simulink model "zumo_control_distance_heading_mod"  (R2014b)
settings: Solver=ode3  SolverMode=SingleTasking  StartTime=0.0  StopTime=20  FixedStep=0.01  RelTol=1e-3
PreLoadFcn:
  | evalin('base','sim=1;');
  | evalin('base','control=0;');
  | evalin('base','bluetoothComm=0;');
  | prepareCurrentFolderForZumo;
  | load MagnetometerBus;
model workspace (MAT data in the model file):
  axleLength = Simulink.Parameter
  axleLength.Value = 9.8
  axleLength.Description = 'Distance between tire contact points
    | of the two wheels/treads
    | in units of centimeters.'
  axleLength.DataType = 'auto'
  commandPercmPerSecond = Simulink.Parameter
  commandPercmPerSecond.Value = 3.9547
  commandPercmPerSecond.Description = 'Convert units of ''command'' 
    | to units of ''cm/s''.
    | 
    | ''command'' is a value in the range [-256, 255].'
  commandPercmPerSecond.DataType = 'auto'
  symmetrizeMotors = Simulink.Parameter
  symmetrizeMotors.Value = 1
  symmetrizeMotors.Description = 'Scale one of the motor commands down 
    | (not up) to balance the motors. 
    | Once balanced, a value of x sent to either
    | motor will produce the same rate of rotation
    | in both motors.'
  symmetrizeMotors.DataType = 'auto'
  sampleTime = Simulink.Parameter
  sampleTime.Value = 0.01
  sampleTime.Description = 'Sample time (in seconds) of the trajectory simulator.'
  sampleTime.DataType = 'auto'
  commandThreshold = Simulink.Parameter
  commandThreshold.Value = 31.875
  commandThreshold.DataType = 'auto'
  lineThreshold = Simulink.Parameter
  lineThreshold.Value = 500
  lineThreshold.DataType = 'auto'
  velocity = Simulink.Parameter
  velocity.Value = 10
  velocity.Description = 'cm / s'
  velocity.DataType = 'auto'
  waveLength = Simulink.Parameter
  waveLength.Value = 8.6
  waveLength.Description = 'Units of cm.
    | 
    | The following condition must be satisfied: 
    | waveLength > 2*pi * velocity / sqrt(0.5 / sampleTime)
    | 
    | For reference,
    | robotLength = 8.6 cm
    | '
  waveLength.DataType = 'auto'
  compassBias = Simulink.Parameter
  compassBias.Value = 120
  compassBias.DataType = 'auto'
undefined symbols (not defined in the file or in its folder): magnitude
libraries: simulink x7, ZumoBotLib x2, arduinolib x2, etargetslib x2
settings Model: ExtModeTrigDuration=2  Creator=pkasseba  LastModifiedBy=sandip
settings DataIOCC: SignalLoggingSaveFormat=ModelDataLogs
settings OptimizationCC: OptimizeModelRefInitCode=on  LifeSpan=1
settings DebuggingCC: UnderspecifiedInitializationDetection=Classic  MergeDetectMultiDrivingBlocksExec=none  SolverPrmCheckMsg=none  MultiTaskDSMMsg=warning  MultiTaskCondExecSysMsg=none  StateNameClashWarn=warning
settings HardwareCC: ProdBitPerInt=16  ProdBitPerPointer=8  ProdIntDivRoundTo=Zero  ProdEndianess=LittleEndian  ProdWordSize=8  ProdHWDeviceType=Atmel->AVR
settings SFSimCC: SimParseCustomCode=off
settings RTWCC: SystemTargetFile=realtime.tlc  GenerateMakefile=off  TemplateMakefile=realtime.tmf  Description=Run on Target Hardware  RTWVerbose=off  ProcessScript=realtime_make_rtw_hook  IncludeERTFirstTime=on
settings STFCustomTargetCC: TargetLibSuffix=.a  GenerateSampleERTMain=on  ERTCustomFileBanners=on  SupportNonInlinedSFcns=off  SupportVariableSizeSignals=on  MATLABClassNameForMDSCustomization=Simulink.SoftwareTarget.ERTCustomization  GRTInterface=off  SystemTargetFile=realtime.tlc
settings ERTTargetCC: GenerateSampleERTMain=on  ParMdlRefBuildCompliant=off  CompOptLevelCompliant=off  ConcurrentExecutionCompliant=off  CombineOutputUpdateFcns=off  ERTFirstTimeCompliant=off  SupportContinuousTime=on  SupportVariableSizeSignals=on  ModelStepFunctionPrototypeControlCompliant=off  CPPClassGenCompliant=off  ExtModeTransport=3  ExtModeMexFile=ext_serial_win32_comm  ExtModeMexArgs=0 1 9600  InlinedParameterPlacement=NonHierarchical  ERTSrcFileBannerTemplate=realtime_code_template.cgt  ERTHdrFileBannerTemplate=realtime_code_template.cgt  ERTDataSrcFileTemplate=realtime_code_template.cgt  ERTDataHdrFileTemplate=realtime_code_template.cgt  ERTCustomFileTemplate=realtime_file_process.tlc

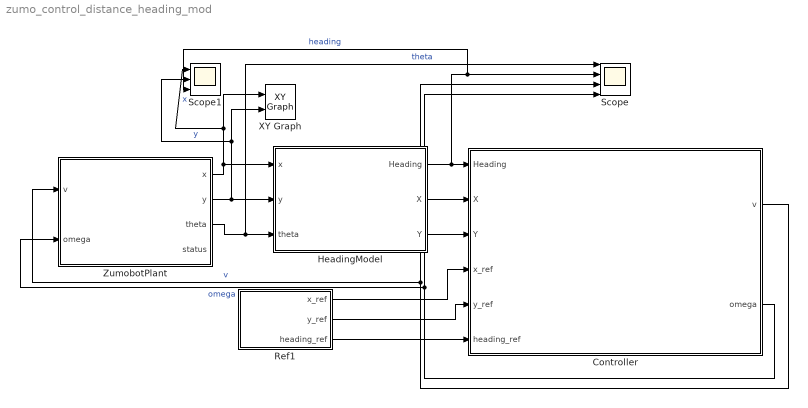
== system zumo_control_distance_heading_mod ==
  Controller : Subsystem
  HeadingModel : Subsystem  Variant=on
  Ref1 : Subsystem
  Scope : Scope  NumInputPorts=4
      settings: TimeRange=0.768348623853211  YMin=-2.5~184~14~-1  YMax=0~186.5~16~1  SaveName=ScopeData4
  Scope1 : Scope  NumInputPorts=3
      settings: YMin=180~100~0  YMax=340~240~350  SaveName=ScopeData2
  XY Graph : simulink/Sinks/XY Graph  xmin=-10  xmax=400  ymin=-10  ymax=400  st=-1
  ZumobotPlant : Subsystem  Variant=on
  wires:
  Controller/1(v) -> Scope/3, ZumobotPlant/1(v)  "v"
  Controller/2(omega) -> Scope/4, ZumobotPlant/2(omega)  "omega"
  ZumobotPlant/3(theta) -> Scope/1, HeadingModel/3(theta)  "theta"
  HeadingModel/2(X) -> Controller/2(X)
  HeadingModel/3(Y) -> Controller/3(Y)
  ZumobotPlant/1(x) -> Scope1/1, XY Graph/1, HeadingModel/1(x)  "x"
  ZumobotPlant/2(y) -> Scope1/2, XY Graph/2, HeadingModel/2(y)  "y"
  HeadingModel/1(Heading) -> Scope1/3, Scope/2, Controller/1(Heading)  "heading"
  Ref1/1(x_ref) -> Controller/4(x_ref)
  Ref1/2(y_ref) -> Controller/5(y_ref)
  Ref1/3(heading_ref) -> Controller/6(heading_ref)

== system zumo_control_distance_heading_mod/Controller ==
  Heading : Inport
  X : Inport  Port=2
  Y : Inport  Port=3
  x_ref : Inport  Port=4
  y_ref : Inport  Port=5
  heading_ref : Inport  Port=6
  Subsystem : Subsystem  Commented=on
  Subsystem1 : Subsystem  Commented=on
  Variant Subsystem : Subsystem  Variant=on
  v : Outport  InitialOutput=0
  omega : Outport  Port=2  InitialOutput=0
  wires:
  Y/1 -> Variant Subsystem/2(Y)
  Heading/1 -> Variant Subsystem/6(Heading)
  Variant Subsystem/1(v) -> v/1
  Variant Subsystem/2(omega) -> omega/1
  X/1 -> Variant Subsystem/1(X)
  x_ref/1 -> Variant Subsystem/3(DesiredX)
  y_ref/1 -> Variant Subsystem/4(DesiredY)
  heading_ref/1 -> Variant Subsystem/5(DesiredHeading)

== system zumo_control_distance_heading_mod/HeadingModel ==
  note: 1) Only subsystems can be added as variant choices at this level
      | 2) Blocks cannot be connected at this level as connectivity is
      | automatically determined at simulation, based on the active variant
  x : Inport
  y : Inport  Port=2
  theta : Inport  Port=3
  Simulation : Subsystem  VariantControl=sim==1
  Target : Subsystem  VariantControl=sim==0
  Heading : Outport
  X : Outport  Port=2
  Y : Outport  Port=3

== system zumo_control_distance_heading_mod/Ref1 ==
  DesiredHeading : Constant  Value=120
  DesiredX : Constant  Value=320
  DesiredY : Constant  Value=240
  x_ref : Outport
  y_ref : Outport  Port=2
  heading_ref : Outport  Port=3
  wires:
  DesiredX/1 -> x_ref/1
  DesiredY/1 -> y_ref/1
  DesiredHeading/1 -> heading_ref/1

== system zumo_control_distance_heading_mod/ZumobotPlant ==
  note: 1) Only subsystems can be added as variant choices at this level
      | 2) Blocks cannot be connected at this level as connectivity is
      | automatically determined at simulation, based on the active variant
  v : Inport
  omega : Inport  Port=2
  Simulation : Subsystem  VariantControl=sim==1
  Target : Subsystem  VariantControl=sim==0
  x : Outport
  y : Outport  Port=2
  theta : Outport  Port=3
  status : Outport  Port=4

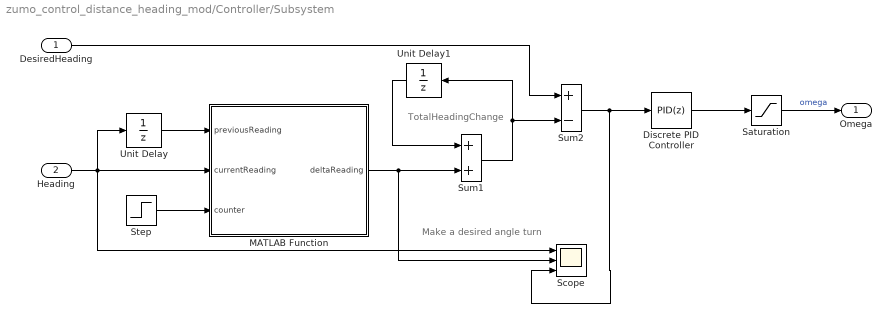
== system zumo_control_distance_heading_mod/Controller/Subsystem ==
  note: Make a desired angle turn
  note: TotalHeadingChange
  DesiredHeading : Inport
  Heading : Inport  Port=2
  Discrete PID Controller : simulink/Continuous/PID Controller  Controller=PID  TimeDomain=Discrete-time  SampleTime=0.01  IntegratorMethod=Forward Euler  FilterMethod=Forward Euler  Form=Parallel  P=20  I=0  D=0  N=100  InitialConditionSource=internal  InitialConditionForIntegrator=0  InitialConditionForFilter=0  ExternalReset=none  LimitOutput=off  UpperSaturationLimit=inf  LowerSaturationLimit=-inf  LinearizeAsGain=off  AntiWindupMode=none  Kb=1  TrackingMode=off  Kt=1  PParamMin=[]  PParamMax=[]  IParamMin=[]  IParamMax=[]  DParamMin=[]  DParamMax=[]  NParamMin=[]  NParamMax=[]  KbParamMin=[]  KbParamMax=[]  KtParamMin=[]  KtParamMax=[]  POutMin=[]  POutMax=[]  IOutMin=[]  IOutMax=[]  DOutMin=[]  DOutMax=[]  NOutMin=[]  NOutMax=[]  KbOutMin=[]  KbOutMax=[]  KtOutMin=[]  KtOutMax=[]  IntegratorOutMin=[]  IntegratorOutMax=[]  FilterOutMin=[]  FilterOutMax=[]  SumOutMin=[]  SumOutMax=[]  SumI1OutMin=[]  SumI1OutMax=[]  SumI2OutMin=[]  SumI2OutMax=[]  SumI3OutMin=[]  SumI3OutMax=[]  SumDOutMin=[]  SumDOutMax=[]  SaturationOutMin=[]  SaturationOutMax=[]  IntegratorContinuousStateAttributes=''  IntegratorStateMustResolveToSignalObject=off  IntegratorRTWStateStorageClass=Auto  FilterContinuousStateAttributes=''  FilterStateMustResolveToSignalObject=off  FilterRTWStateStorageClass=Auto
  MATLAB Function : MATLAB Function  TreatAsAtomicUnit=on
  Saturation : Saturate  UpperLimit=200  LowerLimit=0
  Scope : Scope  NumInputPorts=3
      settings: YMin=266~-1~-4  YMax=266~1~-4
  Step : Step  Time=2*sampleTime  SampleTime=sampleTime
  Sum1 : Sum
  Sum2 : Sum  Inputs=+-
  Unit Delay : UnitDelay  SampleTime=-1
  Unit Delay1 : UnitDelay  SampleTime=-1
  Omega : Outport
  wires:
  Sum1/1 -> Unit Delay1/1, Sum2/2
  Step/1 -> MATLAB Function/3(counter)
  MATLAB Function/1(deltaReading) -> Scope/2, Sum1/2
  Sum2/1 -> Discrete PID Controller/1, Scope/3
  Saturation/1 -> Omega/1  "omega"
  Unit Delay/1 -> MATLAB Function/1(previousReading)
  Unit Delay1/1 -> Sum1/1
  DesiredHeading/1 -> Sum2/1
  Heading/1 -> Unit Delay/1, MATLAB Function/2(currentReading), Scope/1
  Discrete PID Controller/1 -> Saturation/1

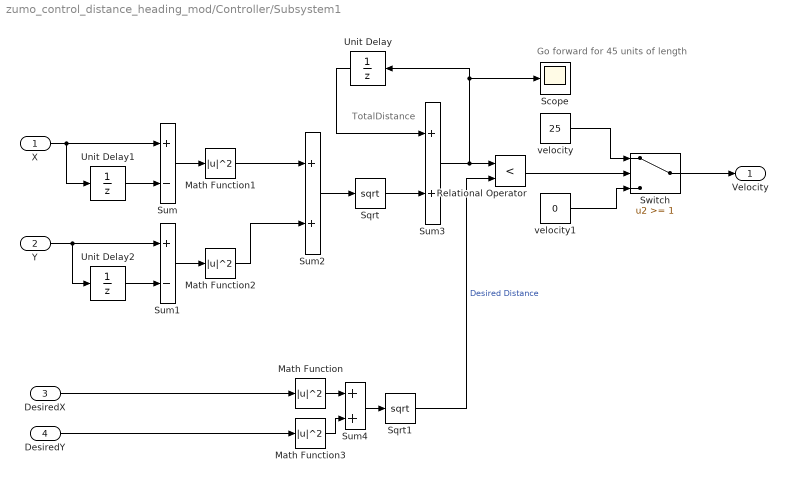
== system zumo_control_distance_heading_mod/Controller/Subsystem1 ==
  note: Go forward for 45 units of length
  note: TotalDistance
  X : Inport
  Y : Inport  Port=2
  DesiredX : Inport  Port=3
  DesiredY : Inport  Port=4
  Math Function{,1..3} (4 alike) : Math  Operator=magnitude^2  SaturateOnIntegerOverflow=on
  Relational Operator : RelationalOperator  Operator=<  OutDataTypeStr=boolean
  Scope : Scope
      settings: YMin=0  YMax=50
  Sqrt : Sqrt  SaturateOnIntegerOverflow=on
  Sqrt1 : Sqrt  SaturateOnIntegerOverflow=on
  Sum : Sum  Inputs=+-
  Sum1 : Sum  Inputs=+-
  Sum2 : Sum
  Sum3 : Sum
  Sum4 : Sum
  Switch : Switch  Threshold=1
  Unit Delay : UnitDelay  SampleTime=-1
  Unit Delay1 : UnitDelay  SampleTime=-1
  Unit Delay2 : UnitDelay  SampleTime=-1
  velocity : Constant  Value=25
  velocity1 : Constant  Value=0
  Velocity : Outport
  wires:
  X/1 -> Unit Delay1/1, Sum/1
  Sqrt/1 -> Sum3/2
  Sum/1 -> Math Function1/1
  Sum2/1 -> Sqrt/1
  Math Function1/1 -> Sum2/1
  velocity/1 -> Switch/1
  Unit Delay1/1 -> Sum/2
  Math Function2/1 -> Sum2/2
  Switch/1 -> Velocity/1
  Sum1/1 -> Math Function2/1
  Unit Delay2/1 -> Sum1/2
  Y/1 -> Unit Delay2/1, Sum1/1
  Unit Delay/1 -> Sum3/1
  Sum3/1 -> Relational Operator/1, Scope/1, Unit Delay/1
  velocity1/1 -> Switch/3
  Relational Operator/1 -> Switch/2
  Math Function3/1 -> Sum4/2
  Math Function/1 -> Sum4/1
  Sum4/1 -> Sqrt1/1
  Sqrt1/1 -> Relational Operator/2  "Desired Distance"
  DesiredX/1 -> Math Function/1
  DesiredY/1 -> Math Function3/1

== system zumo_control_distance_heading_mod/Controller/Variant Subsystem ==
  note: 1) Only subsystems can be added as variant choices at this level
      | 2) Blocks cannot be connected at this level as connectivity is
      | automatically determined at simulation, based on the active variant
  X : Inport
  Y : Inport  Port=2
  DesiredX : Inport  Port=3
  DesiredY : Inport  Port=4
  DesiredHeading : Inport  Port=5
  Heading : Inport  Port=6
  PrimitiveControl : Subsystem  VariantControl=control == 2
  controllyap : MATLAB Function  TreatAsAtomicUnit=on  VariantControl=control==0
  wmr : MATLAB Function  TreatAsAtomicUnit=on  VariantControl=control==1
  v : Outport
  omega : Outport  Port=2

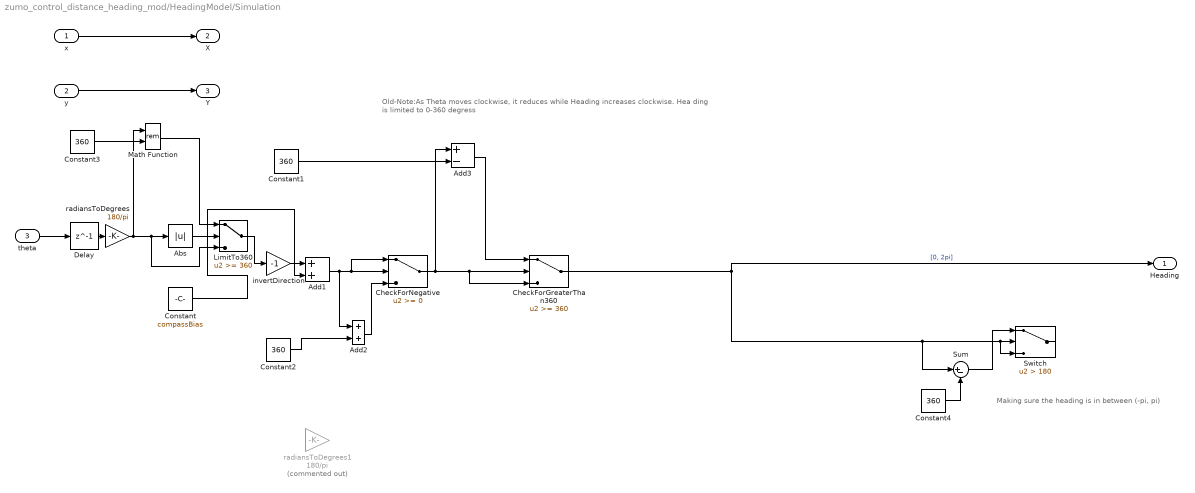
== system zumo_control_distance_heading_mod/HeadingModel/Simulation ==
  note: Old-Note:As Theta moves clockwise, it reduces while Heading increases clockwise.
      | Hea ding is limited to 0-360 degress
  note: Making sure the heading is in between (-pi, pi)
  x : Inport
  y : Inport  Port=2
  theta : Inport  Port=3
  Abs : Abs
  Add1 : Sum
  Add2 : Sum
  Add3 : Sum  Inputs=+-
  CheckForGreaterThan360 : Switch  Threshold=360
  CheckForNegative : Switch
  Constant : Constant  Value=compassBias
  Constant{1..4} (4 alike) : Constant  Value=360
  Delay : Delay  DelayLength=1  InitialCondition=0  SampleTime=sampleTime
  LimitTo360 : Switch  Threshold=360
  Math Function : Math  Operator=rem  SaturateOnIntegerOverflow=on
  Sum : Sum  Inputs=|+-
  Switch : Switch  Criteria=u2 > Threshold  Threshold=180
  invertDirection : Gain  Gain=-1
  radiansToDegrees : Gain  Gain=180/pi
  radiansToDegrees1 : Gain  Commented=on  Gain=180/pi
  Heading : Outport
  X : Outport  Port=2
  Y : Outport  Port=3
  wires:
  x/1 -> X/1
  y/1 -> Y/1
  Delay/1 -> radiansToDegrees/1
  Constant/1 -> Add1/2
  Constant1/1 -> Add3/2
  Add3/1 -> CheckForGreaterThan360/1
  invertDirection/1 -> Add1/1
  Add1/1 -> Add2/1, CheckForNegative/2, CheckForNegative/1
  CheckForNegative/1 -> CheckForGreaterThan360/3, CheckForGreaterThan360/2, Add3/1
  Constant2/1 -> Add2/2
  Add2/1 -> CheckForNegative/3
  radiansToDegrees/1 -> Math Function/1, LimitTo360/3, Abs/1
  LimitTo360/1 -> invertDirection/1
  Constant3/1 -> Math Function/2
  Math Function/1 -> LimitTo360/1
  Abs/1 -> LimitTo360/2
  CheckForGreaterThan360/1 -> Sum/1, Switch/3, Switch/2, Heading/1  "[0, 2pi]"
  Constant4/1 -> Sum/2
  theta/1 -> Delay/1
  Sum/1 -> Switch/1

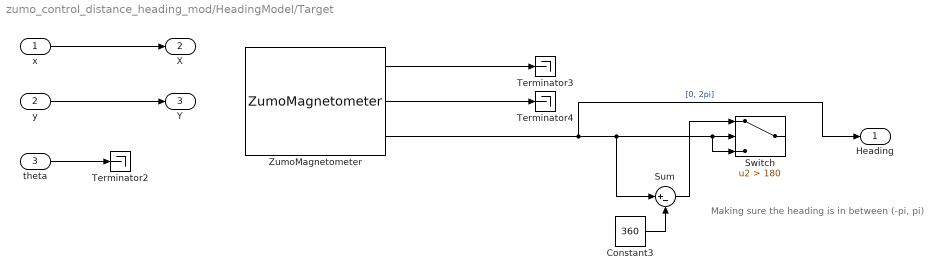
== system zumo_control_distance_heading_mod/HeadingModel/Target ==
  note: Making sure the heading is in between (-pi, pi)
  x : Inport
  y : Inport  Port=2
  theta : Inport  Port=3
  Constant3 : Constant  Value=360
  Sum : Sum  Inputs=|+-
  Switch : Switch  Criteria=u2 > Threshold  Threshold=180
  Terminator2 : Terminator
  Terminator3 : Terminator
  Terminator4 : Terminator
  ZumoMagnetometer : ZumoBotLib/ZumoMagnetometer  sampletime_lsm=0.01  debug_lsm=off  minX_lsm=-512  maxX_lsm=-279  minY_lsm=-163  maxY_lsm=99  minZ_lsm=1302  maxZ_lsm=1580
      link override S-Function Builder: Parameters=sampletime_lsm,boolean(debug_lsm),minX_lsm,maxX_lsm,minY_lsm,maxY_lsm,minZ_lsm,boolean(maxZ_lsm)
  Heading : Outport
  X : Outport  Port=2
  Y : Outport  Port=3
  wires:
  x/1 -> X/1
  y/1 -> Y/1
  theta/1 -> Terminator2/1
  ZumoMagnetometer/1 -> Terminator3/1
  ZumoMagnetometer/2 -> Terminator4/1
  ZumoMagnetometer/3 -> Heading/1, Sum/1, Switch/3, Switch/2  "[0, 2pi]"
  Constant3/1 -> Sum/2
  Sum/1 -> Switch/1

== system zumo_control_distance_heading_mod/ZumobotPlant/Simulation ==
  v : Inport
  omega : Inport  Port=2
  Computation of x,y,theta : Subsystem  Variant=on  OverrideUsingVariant=bluetoothComm==0
  Delay : Delay  DelayLength=1  InitialCondition=0
  degreesToRadians : Gain  Gain=pi/180
  motor command conversion : Subsystem
  x : Outport
  y : Outport  Port=2
  theta : Outport  Port=3
  status : Outport  Port=4
  wires:
  v/1 -> motor command conversion/1(v)
  Computation of x,y,theta/1(x) -> x/1
  Computation of x,y,theta/2(y) -> y/1
  omega/1 -> degreesToRadians/1
  Computation of x,y,theta/3(theta) -> theta/1
  degreesToRadians/1 -> motor command conversion/2(omega)
  motor command conversion/1(v_L v_R) -> Delay/1
  Delay/1 -> Computation of x,y,theta/1(v_L v_R)

== system zumo_control_distance_heading_mod/ZumobotPlant/Target ==
  v : Inport
  omega : Inport  Port=2
  Computation of x,y,theta : Subsystem  Variant=on  OverrideUsingVariant=bluetoothComm==1
  Demux : Demux  Outputs=2
  ZumoMotors : ZumoBotLib/ZumoMotors  flipLeft=off  flipRight=off
  degreesToRadians : Gain  Gain=pi/180
  motor command conversion : Subsystem
  x : Outport
  y : Outport  Port=2
  theta : Outport  Port=3
  status : Outport  Port=4
  wires:
  motor command conversion/1(v_L v_R) -> Computation of x,y,theta/1(v_L v_R), Demux/1
  Demux/1 -> ZumoMotors/1
  Demux/2 -> ZumoMotors/2
  v/1 -> motor command conversion/1(v)
  omega/1 -> degreesToRadians/1
  degreesToRadians/1 -> motor command conversion/2(omega)
  Computation of x,y,theta/1(x) -> x/1
  Computation of x,y,theta/2(y) -> y/1
  Computation of x,y,theta/3(theta) -> theta/1
  Computation of x,y,theta/4(status) -> status/1

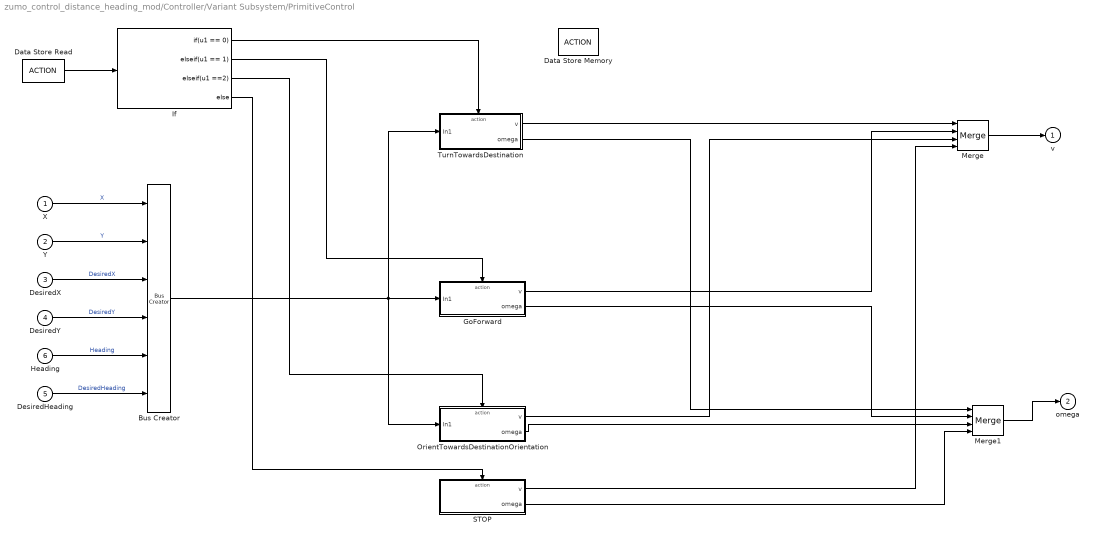
== system zumo_control_distance_heading_mod/Controller/Variant Subsystem/PrimitiveControl ==
  X : Inport
  Y : Inport  Port=2
  DesiredX : Inport  Port=3
  DesiredY : Inport  Port=4
  DesiredHeading : Inport  Port=5
  Heading : Inport  Port=6
  Bus Creator : BusCreator  Inputs=6
  Data Store Memory : DataStoreMemory  DataStoreName=ACTION  ReadBeforeWriteMsg=warning  WriteAfterWriteMsg=warning  WriteAfterReadMsg=warning
  Data Store Read : DataStoreRead  DialogController=Simulink.DDGSource  DataStoreName=ACTION  SampleTime=sampleTime  DataStoreElements=ACTION
  GoForward : Subsystem  TreatAsAtomicUnit=on
  If : If  IfExpression=u1 == 0  ElseIfExpressions=u1 == 1, u1 ==2
  Merge : Merge  Inputs=4
  Merge1 : Merge  Inputs=4
  OrientTowardsDestinationOrientation : Subsystem  TreatAsAtomicUnit=on
  STOP : Subsystem  TreatAsAtomicUnit=on
  TurnTowardsDestination : Subsystem  TreatAsAtomicUnit=on
  v : Outport
  omega : Outport  Port=2
  wires:
  X/1 -> Bus Creator/1  "X"
  Y/1 -> Bus Creator/2  "Y"
  DesiredX/1 -> Bus Creator/3  "DesiredX"
  DesiredY/1 -> Bus Creator/4  "DesiredY"
  DesiredHeading/1 -> Bus Creator/6  "DesiredHeading"
  Heading/1 -> Bus Creator/5  "Heading"
  Data Store Read/1 -> If/1
  If/1 -> TurnTowardsDestination/Action
  If/2 -> GoForward/Action
  If/3 -> OrientTowardsDestinationOrientation/Action
  Merge/1 -> v/1
  Merge1/1 -> omega/1
  TurnTowardsDestination/1(v) -> Merge/1
  GoForward/1(v) -> Merge/2
  OrientTowardsDestinationOrientation/1(v) -> Merge/3
  TurnTowardsDestination/2(omega) -> Merge1/1
  OrientTowardsDestinationOrientation/2(omega) -> Merge1/3
  GoForward/2(omega) -> Merge1/2
  Bus Creator/1 -> OrientTowardsDestinationOrientation/1(In1), TurnTowardsDestination/1(In1), GoForward/1(In1)
  STOP/1(v) -> Merge/4
  STOP/2(omega) -> Merge1/4
  If/4 -> STOP/Action

== system zumo_control_distance_heading_mod/ZumobotPlant/Simulation/Computation of x,y,theta ==
  note: 1) Only subsystems can be added as variant choices at this level
      | 2) Blocks cannot be connected at this level as connectivity is
      | automatically determined at simulation, based on the active variant
  v_L v_R : Inport
  simulated trajectory/ replacing encoders : Subsystem  VariantControl=bluetoothComm==0
  "values from bluetooth " : Subsystem  VariantControl=bluetoothComm==1
  x : Outport
  y : Outport  Port=2
  theta : Outport  Port=3

== system zumo_control_distance_heading_mod/ZumobotPlant/Simulation/motor command conversion ==
  note: or in matrix notation,
  note: v_L  = v - omega * axleLength/2
      | v_R = v + omega * axleLength/2
  note: [v_L; v_R] = [1 -axleLength/2; 1 axleLength/2] * [v; omega]
  v : Inport
  omega : Inport  Port=2
  Mux : Mux  Inputs=2
  Saturation [-256 255] : Saturate  UpperLimit=255  LowerLimit=-256
  change parameters : Gain  Gain=[1 -axleLength/2; 1 axleLength/2]  Multiplication=Matrix(K*u)
  change units : Gain  Gain=commandPercmPerSecond
  symmetrize motors : Gain  Gain=[1 symmetrizeMotors]
  v_L v_R : Outport
  wires:
  change parameters/1 -> symmetrize motors/1  "v_L v_R"
  change units/1 -> Saturation [-256 255]/1  "v_L v_R (command)"
  symmetrize motors/1 -> change units/1  "v_L v_R (cm/s)"
  Saturation [-256 255]/1 -> v_L v_R/1
  Mux/1 -> change parameters/1
  omega/1 -> Mux/2
  v/1 -> Mux/1

== system zumo_control_distance_heading_mod/ZumobotPlant/Target/Computation of x,y,theta ==
  note: 1) Only subsystems can be added as variant choices at this level
      | 2) Blocks cannot be connected at this level as connectivity is
      | automatically determined at simulation, based on the active variant
  v_L v_R : Inport
  simulated trajectory/ replacing encoders : Subsystem  VariantControl=bluetoothComm==0
  "values from bluetooth " : Subsystem  VariantControl=bluetoothComm==1
  x : Outport
  y : Outport  Port=2
  theta : Outport  Port=3
  status : Outport  Port=4

== system zumo_control_distance_heading_mod/ZumobotPlant/Target/motor command conversion ==
  note: or in matrix notation,
  note: v_L  = v - omega * axleLength/2
      | v_R = v + omega * axleLength/2
  note: [v_L; v_R] = [1 -axleLength/2; 1 axleLength/2] * [v; omega]
  v : Inport
  omega : Inport  Port=2
  Mux : Mux  Inputs=2
  Saturation [-256 255] : Saturate  UpperLimit=255  LowerLimit=-256
  change parameters : Gain  Gain=[1 -axleLength/2; 1 axleLength/2]  Multiplication=Matrix(K*u)
  change units : Gain  Gain=commandPercmPerSecond
  scaling to +/-50 : Lookup_n-D  Commented=through  NumberOfTableDimensions=1  BreakpointsForDimension1=[-500 -256 255 500]  Table=[-70 -70 70 70]  ExtrapMethod=Clip  InternalRulePriority=Speed  RndMeth=Simplest  InputSameDT=on
  symmetrize motors : Gain  Gain=[1 symmetrizeMotors]
  v_L v_R : Outport
  wires:
  change parameters/1 -> symmetrize motors/1  "v_L v_R"
  change units/1 -> Saturation [-256 255]/1  "v_L v_R (command)"
  symmetrize motors/1 -> change units/1  "v_L v_R (cm/s)"
  Saturation [-256 255]/1 -> scaling to +/-50/1
  Mux/1 -> change parameters/1
  omega/1 -> Mux/2
  v/1 -> Mux/1
  scaling to +/-50/1 -> v_L v_R/1

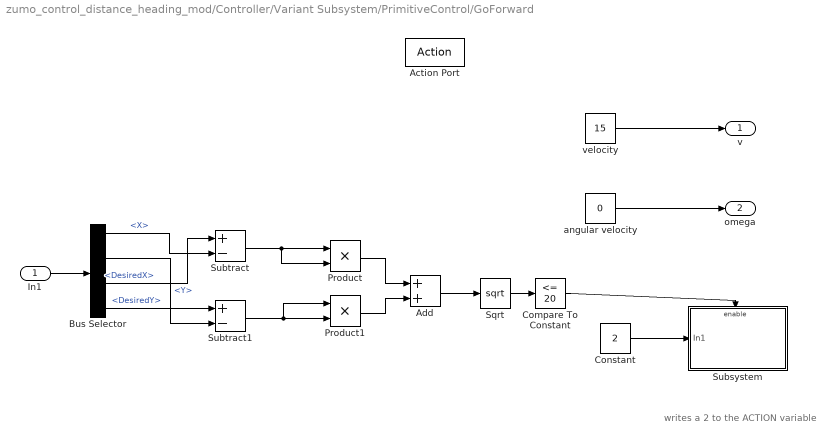
== system zumo_control_distance_heading_mod/Controller/Variant Subsystem/PrimitiveControl/GoForward ==
  note: writes a 2 to the ACTION variable
  In1 : Inport
  Action Port : ActionPort  ActionType=elseif
  Add : Sum
  Bus Selector : BusSelector  OutputSignals=X,Y,DesiredX,DesiredY
  Compare To Constant : simulink/Logic and Bit Operations/Compare To Constant  relop=<=  const=20  OutDataTypeStr=boolean
  Constant : Constant  Value=2
  Product : Product
  Product1 : Product
  Sqrt : Sqrt  SaturateOnIntegerOverflow=on
  Subsystem : Subsystem
  Subtract : Sum  Inputs=+-
  Subtract1 : Sum  Inputs=+-
  angular velocity : Constant  Value=0
  velocity : Constant  Value=15
  v : Outport  InitialOutput=0
  omega : Outport  Port=2  InitialOutput=0
  wires:
  angular velocity/1 -> omega/1
  velocity/1 -> v/1
  In1/1 -> Bus Selector/1
  Add/1 -> Sqrt/1
  Product/1 -> Add/1
  Product1/1 -> Add/2
  Subtract/1 -> Product/2, Product/1
  Subtract1/1 -> Product1/2, Product1/1
  Bus Selector/1 -> Subtract/2  "<X>"
  Bus Selector/3 -> Subtract/1  "<DesiredX>"
  Bus Selector/2 -> Subtract1/2  "<Y>"
  Bus Selector/4 -> Subtract1/1  "<DesiredY>"
  Sqrt/1 -> Compare To Constant/1
  Compare To Constant/1 -> Subsystem/Enable
  Constant/1 -> Subsystem/1(In1)

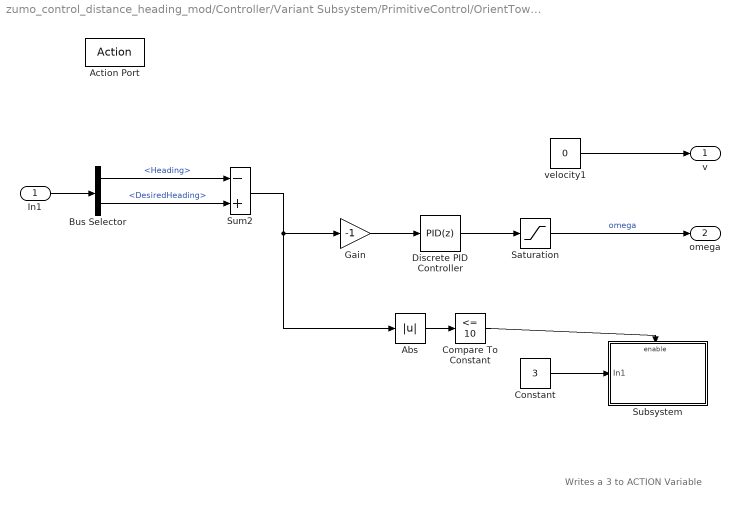
== system zumo_control_distance_heading_mod/Controller/Variant Subsystem/PrimitiveControl/OrientTowardsDestinationOrientation ==
  note: Writes a 3 to ACTION Variable
  In1 : Inport
  Action Port : ActionPort  ActionType=elseif
  Abs : Abs
  Bus Selector : BusSelector  OutputSignals=Heading,DesiredHeading
  Compare To Constant : simulink/Logic and Bit Operations/Compare To Constant  relop=<=  const=10  OutDataTypeStr=boolean
  Constant : Constant  Value=3
  Discrete PID Controller : simulink/Continuous/PID Controller  Controller=PID  TimeDomain=Discrete-time  SampleTime=0.01  IntegratorMethod=Forward Euler  FilterMethod=Forward Euler  Form=Parallel  P=100  I=0  D=0  N=100  InitialConditionSource=internal  InitialConditionForIntegrator=0  InitialConditionForFilter=0  ExternalReset=none  LimitOutput=off  UpperSaturationLimit=inf  LowerSaturationLimit=-inf  LinearizeAsGain=off  AntiWindupMode=none  Kb=1  TrackingMode=off  Kt=1  PParamMin=[]  PParamMax=[]  IParamMin=[]  IParamMax=[]  DParamMin=[]  DParamMax=[]  NParamMin=[]  NParamMax=[]  KbParamMin=[]  KbParamMax=[]  KtParamMin=[]  KtParamMax=[]  POutMin=[]  POutMax=[]  IOutMin=[]  IOutMax=[]  DOutMin=[]  DOutMax=[]  NOutMin=[]  NOutMax=[]  KbOutMin=[]  KbOutMax=[]  KtOutMin=[]  KtOutMax=[]  IntegratorOutMin=[]  IntegratorOutMax=[]  FilterOutMin=[]  FilterOutMax=[]  SumOutMin=[]  SumOutMax=[]  SumI1OutMin=[]  SumI1OutMax=[]  SumI2OutMin=[]  SumI2OutMax=[]  SumI3OutMin=[]  SumI3OutMax=[]  SumDOutMin=[]  SumDOutMax=[]  SaturationOutMin=[]  SaturationOutMax=[]  IntegratorContinuousStateAttributes=''  IntegratorStateMustResolveToSignalObject=off  IntegratorRTWStateStorageClass=Auto  FilterContinuousStateAttributes=''  FilterStateMustResolveToSignalObject=off  FilterRTWStateStorageClass=Auto  DifferentiatorICPrevScaledInput=0  DifferentiatorOutMin=[]  DifferentiatorOutMax=[]  UseFilter=on
  Gain : Gain  Gain=-1
  Saturation : Saturate  UpperLimit=100  LowerLimit=-100
  Subsystem : Subsystem
  Sum2 : Sum  Inputs=-+
  velocity1 : Constant  Value=0
  v : Outport
  omega : Outport  Port=2
  wires:
  In1/1 -> Bus Selector/1
  velocity1/1 -> v/1
  Bus Selector/2 -> Sum2/2  "<DesiredHeading>"
  Sum2/1 -> Abs/1, Gain/1
  Saturation/1 -> omega/1  "omega"
  Bus Selector/1 -> Sum2/1  "<Heading>"
  Discrete PID Controller/1 -> Saturation/1
  Abs/1 -> Compare To Constant/1
  Compare To Constant/1 -> Subsystem/Enable
  Constant/1 -> Subsystem/1(In1)
  Gain/1 -> Discrete PID Controller/1

== system zumo_control_distance_heading_mod/Controller/Variant Subsystem/PrimitiveControl/STOP ==
  Action Port : ActionPort  ActionType=else
  velocity1 : Constant  Value=0
  velocity2 : Constant  Value=0
  v : Outport
  omega : Outport  Port=2
  wires:
  velocity1/1 -> v/1
  velocity2/1 -> omega/1

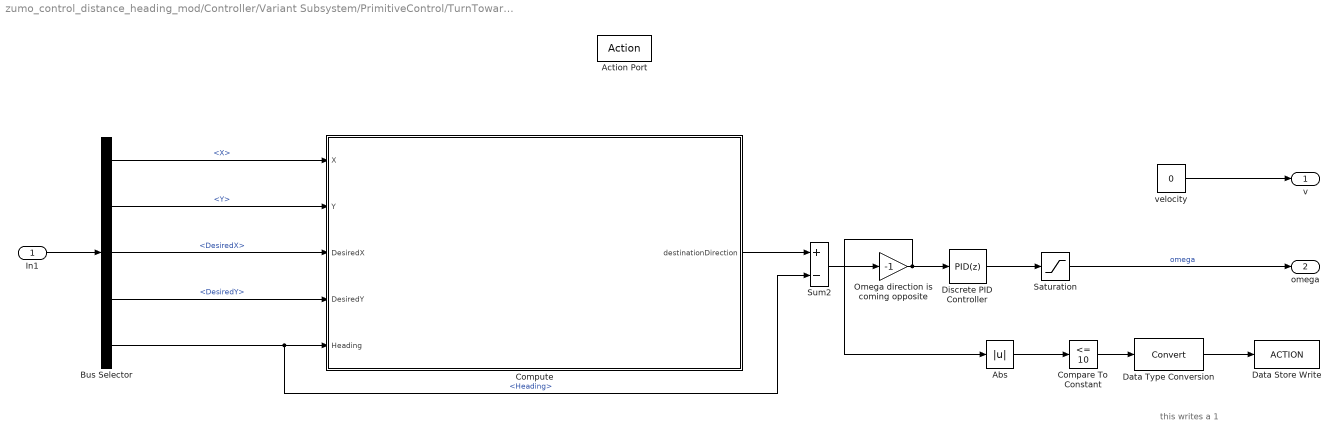
== system zumo_control_distance_heading_mod/Controller/Variant Subsystem/PrimitiveControl/TurnTowardsDestination ==
  note: this writes a 1
  In1 : Inport
  Action Port : ActionPort  ActionType=then
  Abs : Abs
  Bus Selector : BusSelector  OutputSignals=X,Y,DesiredX,DesiredY,Heading
  Compare To Constant : simulink/Logic and Bit Operations/Compare To Constant  relop=<=  const=10  OutDataTypeStr=boolean
  Compute : MATLAB Function  TreatAsAtomicUnit=on
  Data Store Write : DataStoreWrite  DialogController=Simulink.DDGSource  DataStoreName=ACTION  DataStoreElements=ACTION
  Data Type Conversion : DataTypeConversion
  Discrete PID Controller : simulink/Continuous/PID Controller  Controller=PID  TimeDomain=Discrete-time  SampleTime=0.01  IntegratorMethod=Forward Euler  FilterMethod=Forward Euler  Form=Parallel  P=100  I=0  D=0  N=100  InitialConditionSource=internal  InitialConditionForIntegrator=0  InitialConditionForFilter=0  ExternalReset=none  LimitOutput=off  UpperSaturationLimit=inf  LowerSaturationLimit=-inf  LinearizeAsGain=off  AntiWindupMode=none  Kb=1  TrackingMode=off  Kt=1  PParamMin=[]  PParamMax=[]  IParamMin=[]  IParamMax=[]  DParamMin=[]  DParamMax=[]  NParamMin=[]  NParamMax=[]  KbParamMin=[]  KbParamMax=[]  KtParamMin=[]  KtParamMax=[]  POutMin=[]  POutMax=[]  IOutMin=[]  IOutMax=[]  DOutMin=[]  DOutMax=[]  NOutMin=[]  NOutMax=[]  KbOutMin=[]  KbOutMax=[]  KtOutMin=[]  KtOutMax=[]  IntegratorOutMin=[]  IntegratorOutMax=[]  FilterOutMin=[]  FilterOutMax=[]  SumOutMin=[]  SumOutMax=[]  SumI1OutMin=[]  SumI1OutMax=[]  SumI2OutMin=[]  SumI2OutMax=[]  SumI3OutMin=[]  SumI3OutMax=[]  SumDOutMin=[]  SumDOutMax=[]  SaturationOutMin=[]  SaturationOutMax=[]  IntegratorContinuousStateAttributes=''  IntegratorStateMustResolveToSignalObject=off  IntegratorRTWStateStorageClass=Auto  FilterContinuousStateAttributes=''  FilterStateMustResolveToSignalObject=off  FilterRTWStateStorageClass=Auto  DifferentiatorICPrevScaledInput=0  DifferentiatorOutMin=[]  DifferentiatorOutMax=[]  UseFilter=on
  Omega direction is coming opposite : Gain  Gain=-1
  Saturation : Saturate  UpperLimit=100  LowerLimit=-100
  Sum2 : Sum  Inputs=+-
  velocity : Constant  Value=0
  v : Outport  InitialOutput=0
  omega : Outport  Port=2
  wires:
  velocity/1 -> v/1
  In1/1 -> Bus Selector/1
  Bus Selector/1 -> Compute/1(X)  "<X>"
  Bus Selector/2 -> Compute/2(Y)  "<Y>"
  Bus Selector/3 -> Compute/3(DesiredX)  "<DesiredX>"
  Bus Selector/4 -> Compute/4(DesiredY)  "<DesiredY>"
  Bus Selector/5 -> Sum2/2, Compute/5(Heading)  "<Heading>"
  Sum2/1 -> Omega direction is coming opposite/1
  Saturation/1 -> omega/1  "omega"
  Compute/1(destinationDirection) -> Sum2/1
  Discrete PID Controller/1 -> Saturation/1
  Abs/1 -> Compare To Constant/1
  Compare To Constant/1 -> Data Type Conversion/1
  Data Type Conversion/1 -> Data Store Write/1
  Omega direction is coming opposite/1 -> Abs/1, Discrete PID Controller/1

== system zumo_control_distance_heading_mod/ZumobotPlant/Simulation/Computation of x,y,theta/simulated trajectory// replacing encoders ==
  v_L v_R : Inport
  Delay : Delay  DelayLength=1  InitialCondition=0
  Demux : Demux  Outputs=2
  Effective Motor Command : Subsystem
  Scope : Scope  NumInputPorts=2
      settings: YMin=-1~0.188496  YMax=1~0.188496  SaveName=ScopeData3
  calculate simulated trajectory1 : Subsystem
  change parameters : Gain  Gain=[0.5 0.5; -1/axleLength 1/axleLength]  Multiplication=Matrix(K*u)
  change units : Gain  Gain=1/commandPercmPerSecond
  x : Outport
  y : Outport  Port=2
  theta : Outport  Port=3
  wires:
  Demux/2 -> Scope/1, calculate simulated trajectory1/2(omega)
  Demux/1 -> calculate simulated trajectory1/1(v)
  v_L v_R/1 -> Delay/1
  Effective Motor Command/1(c_eff) -> change units/1  "v_L v_R (command)"
  change units/1 -> change parameters/1  "v_L v_R (cm/s)"
  change parameters/1 -> Demux/1  "v omega"
  calculate simulated trajectory1/2(y) -> y/1
  calculate simulated trajectory1/1(x) -> x/1
  calculate simulated trajectory1/3(theta) -> Scope/2, theta/1
  Delay/1 -> Effective Motor Command/1(c)

== system zumo_control_distance_heading_mod/ZumobotPlant/Simulation/Computation of x,y,theta/values from bluetooth  ==
  v_L v_R : Inport
  Serial Receive : arduinolib/Serial Receive  portNumber=0  showOutStatus=on  sampleTime=1  blockPlatform=arduino
  Subsystem : Subsystem
  Subsystem1 : Subsystem
  Terminator : Terminator
  x : Outport
  y : Outport  Port=2
  theta : Outport  Port=3
  wires:
  v_L v_R/1 -> Terminator/1
  Subsystem/1(Out1) -> x/1
  Subsystem/2(Out2) -> y/1
  Subsystem/3(Out3) -> theta/1
  Serial Receive/1 -> Subsystem1/1(In1)  "[x,y]"
  Subsystem1/1(Out1) -> Subsystem/1(In1)
  Subsystem1/2(status) -> Subsystem/Trigger
  Serial Receive/2 -> Subsystem1/Trigger

== system zumo_control_distance_heading_mod/ZumobotPlant/Target/Computation of x,y,theta/simulated trajectory// replacing encoders ==
  v_L v_R : Inport
  Delay : Delay  DelayLength=1  InitialCondition=0
  Demux : Demux  Outputs=2
  Effective Motor Command : Subsystem
  Scope : Scope  NumInputPorts=2
      settings: YMin=-1~0.188496  YMax=1~0.188496  SaveName=ScopeData3
  calculate simulated trajectory1 : Subsystem
  change parameters : Gain  Gain=[0.5 0.5; -1/axleLength 1/axleLength]  Multiplication=Matrix(K*u)
  change units : Gain  Gain=1/commandPercmPerSecond
  x : Outport
  y : Outport  Port=2
  theta : Outport  Port=3
  status : Outport  Port=4
  wires:
  Demux/2 -> Scope/1, calculate simulated trajectory1/2(omega)
  Demux/1 -> calculate simulated trajectory1/1(v)
  v_L v_R/1 -> Delay/1
  Effective Motor Command/1(c_eff) -> change units/1  "v_L v_R (command)"
  change units/1 -> change parameters/1  "v_L v_R (cm/s)"
  change parameters/1 -> Demux/1  "v omega"
  calculate simulated trajectory1/2(y) -> y/1
  calculate simulated trajectory1/1(x) -> x/1
  calculate simulated trajectory1/3(theta) -> Scope/2, theta/1
  Delay/1 -> Effective Motor Command/1(c)

== system zumo_control_distance_heading_mod/ZumobotPlant/Target/Computation of x,y,theta/values from bluetooth  ==
  v_L v_R : Inport
  Serial Receive : arduinolib/Serial Receive  portNumber=0  showOutStatus=on  sampleTime=0.01  blockPlatform=arduino
  Subsystem : Subsystem
  Subsystem1 : Subsystem
  Terminator : Terminator
  x : Outport
  y : Outport  Port=2
  theta : Outport  Port=3
  status : Outport  Port=4
  wires:
  v_L v_R/1 -> Terminator/1
  Subsystem/3(theta) -> theta/1
  Serial Receive/1 -> Subsystem1/1(In1)  "[x,y]"
  Subsystem1/1(Out1) -> Subsystem/1(In1)
  Subsystem/1(x) -> x/1
  Subsystem/2(y) -> y/1
  Subsystem1/2(status) -> Subsystem/Enable, status/1
  Serial Receive/2 -> Subsystem1/Enable

== system zumo_control_distance_heading_mod/Controller/Variant Subsystem/PrimitiveControl/GoForward/Subsystem ==
  In1 : Inport
  Enable : EnablePort
  Data Store Write : DataStoreWrite  DialogController=Simulink.DDGSource  DataStoreName=ACTION  DataStoreElements=ACTION
  wires:
  In1/1 -> Data Store Write/1

== system zumo_control_distance_heading_mod/Controller/Variant Subsystem/PrimitiveControl/OrientTowardsDestinationOrientation/Subsystem ==
  In1 : Inport
  Enable : EnablePort
  Data Store Write : DataStoreWrite  DialogController=Simulink.DDGSource  DataStoreName=ACTION  DataStoreElements=ACTION
  wires:
  In1/1 -> Data Store Write/1

== system zumo_control_distance_heading_mod/ZumobotPlant/Simulation/Computation of x,y,theta/simulated trajectory// replacing encoders/Effective Motor Command ==
  note: Zumobot does not move when given a command
      | with an abs less than 50 on a smooth surface,
      | so such commands are effectively 0.
  note: Do not saturate this signal.The process of symmetrizing
      | the motor commands gives rise to this artificial signal,
      | which can exceed the value of 255.
  c : Inport
  Abs : Abs
  Constant1 : Constant  Value=0
  Sum : Sum  Inputs=|+-
  Switch : Switch
  command threshold : Constant  Value=commandThreshold
  symmetrize motors : Gain  Gain=[1 1/symmetrizeMotors]
  c_eff : Outport
  wires:
  Switch/1 -> c_eff/1
  symmetrize motors/1 -> Abs/1, Switch/1
  Sum/1 -> Switch/2
  Abs/1 -> Sum/1
  command threshold/1 -> Sum/2
  c/1 -> symmetrize motors/1  "v_L v_R"
  Constant1/1 -> Switch/3

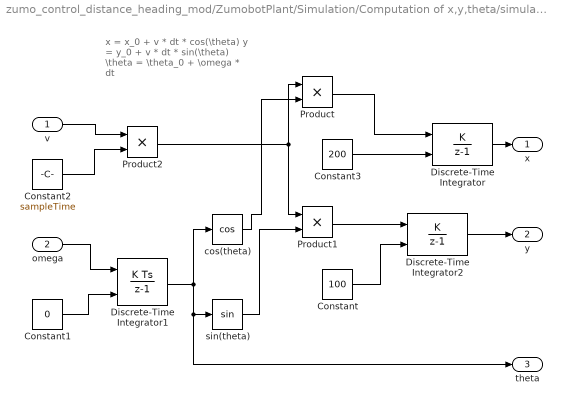
== system zumo_control_distance_heading_mod/ZumobotPlant/Simulation/Computation of x,y,theta/simulated trajectory// replacing encoders/calculate simulated trajectory1 ==
  note: x = x_0 + v * dt * cos(\theta)
      | y = y_0 + v * dt * sin(\theta)
      | \theta = \theta_0 + \omega * dt
  v : Inport
  omega : Inport  Port=2
  Constant : Constant  Value=100
  Constant1 : Constant  Value=0
  Constant2 : Constant  Value=sampleTime
  Constant3 : Constant  Value=200
  Discrete-Time Integrator : DiscreteIntegrator  IntegratorMethod=Accumulation: Forward Euler  InitialConditionSource=external  SampleTime=-1
  Discrete-Time Integrator1 : DiscreteIntegrator  InitialConditionSource=external  SampleTime=-1
  Discrete-Time Integrator2 : DiscreteIntegrator  IntegratorMethod=Accumulation: Forward Euler  InitialConditionSource=external  SampleTime=-1
  Product : Product
  Product1 : Product
  Product2 : Product
  cos(theta) : Trigonometry  Operator=cos
  sin(theta) : Trigonometry
  x : Outport
  y : Outport  Port=2
  theta : Outport  Port=3
  wires:
  omega/1 -> Discrete-Time Integrator1/1
  v/1 -> Product2/1
  Discrete-Time Integrator1/1 -> theta/1, sin(theta)/1, cos(theta)/1
  Product/1 -> Discrete-Time Integrator/1
  cos(theta)/1 -> Product/2
  Product2/1 -> Product/1, Product1/1
  sin(theta)/1 -> Product1/2
  Constant3/1 -> Discrete-Time Integrator/2
  Constant1/1 -> Discrete-Time Integrator1/2
  Constant2/1 -> Product2/2
  Discrete-Time Integrator/1 -> x/1
  Product1/1 -> Discrete-Time Integrator2/1
  Discrete-Time Integrator2/1 -> y/1
  Constant/1 -> Discrete-Time Integrator2/2

== system zumo_control_distance_heading_mod/ZumobotPlant/Simulation/Computation of x,y,theta/values from bluetooth /Subsystem ==
  In1 : Inport
  Trigger : TriggerPort  PortDimensions=1
  Byte Unpack : etargetslib/Byte Unpack  dimensions={1,1}  datatypes={'uint16', 'uint16'}  byteAlign=1
  Fcn : Fcn  Expr=atan2(u(1), u(2))
  Mux : Mux  Inputs=2
  Subtract : Sum  Inputs=+-
  Subtract1 : Sum  Inputs=+-
  Unit Delay : UnitDelay  SampleTime=-1
  Unit Delay1 : UnitDelay  SampleTime=-1
  Out1 : Outport
  Out2 : Outport  Port=2
  Out3 : Outport  Port=3
  wires:
  Byte Unpack/1 -> Unit Delay/1, Out1/1, Subtract/1
  Byte Unpack/2 -> Unit Delay1/1, Out2/1, Subtract1/1
  Subtract1/1 -> Mux/2  "dy"
  Mux/1 -> Fcn/1
  Subtract/1 -> Mux/1  "dx"
  Fcn/1 -> Out3/1
  Unit Delay/1 -> Subtract/2
  Unit Delay1/1 -> Subtract1/2
  In1/1 -> Byte Unpack/1

== system zumo_control_distance_heading_mod/ZumobotPlant/Simulation/Computation of x,y,theta/values from bluetooth /Subsystem1 ==
  In1 : Inport
  Trigger : TriggerPort  PortDimensions=1
  MATLAB Function : MATLAB Function  TreatAsAtomicUnit=on
  Out1 : Outport
  status : Outport  Port=2
  wires:
  In1/1 -> MATLAB Function/1(u)
  MATLAB Function/1(y) -> Out1/1
  MATLAB Function/2(trigger) -> status/1

== system zumo_control_distance_heading_mod/ZumobotPlant/Target/Computation of x,y,theta/simulated trajectory// replacing encoders/Effective Motor Command ==
  note: Zumobot does not move when given a command
      | with an abs less than 50 on a smooth surface,
      | so such commands are effectively 0.
  note: Do not saturate this signal.The process of symmetrizing
      | the motor commands gives rise to this artificial signal,
      | which can exceed the value of 255.
  c : Inport
  Abs : Abs
  Constant1 : Constant  Value=0
  Sum : Sum  Inputs=|+-
  Switch : Switch
  command threshold : Constant  Value=commandThreshold
  symmetrize motors : Gain  Gain=[1 1/symmetrizeMotors]
  c_eff : Outport
  wires:
  Switch/1 -> c_eff/1
  symmetrize motors/1 -> Abs/1, Switch/1
  Sum/1 -> Switch/2
  Abs/1 -> Sum/1
  command threshold/1 -> Sum/2
  c/1 -> symmetrize motors/1  "v_L v_R"
  Constant1/1 -> Switch/3

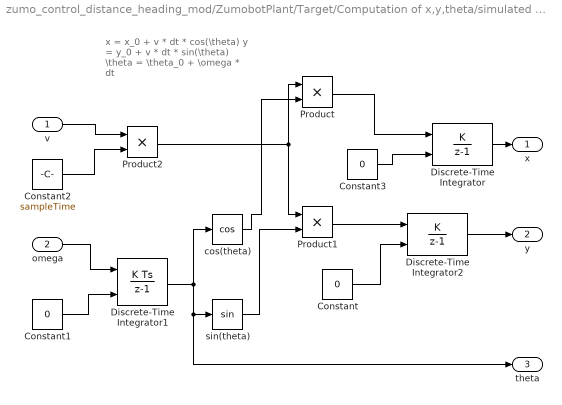
== system zumo_control_distance_heading_mod/ZumobotPlant/Target/Computation of x,y,theta/simulated trajectory// replacing encoders/calculate simulated trajectory1 ==
  note: x = x_0 + v * dt * cos(\theta)
      | y = y_0 + v * dt * sin(\theta)
      | \theta = \theta_0 + \omega * dt
  v : Inport
  omega : Inport  Port=2
  Constant : Constant  Value=0
  Constant1 : Constant  Value=0
  Constant2 : Constant  Value=sampleTime
  Constant3 : Constant  Value=0
  Discrete-Time Integrator : DiscreteIntegrator  IntegratorMethod=Accumulation: Forward Euler  InitialConditionSource=external  SampleTime=-1
  Discrete-Time Integrator1 : DiscreteIntegrator  InitialConditionSource=external  SampleTime=-1
  Discrete-Time Integrator2 : DiscreteIntegrator  IntegratorMethod=Accumulation: Forward Euler  InitialConditionSource=external  SampleTime=-1
  Product : Product
  Product1 : Product
  Product2 : Product
  cos(theta) : Trigonometry  Operator=cos
  sin(theta) : Trigonometry
  x : Outport
  y : Outport  Port=2
  theta : Outport  Port=3
  wires:
  omega/1 -> Discrete-Time Integrator1/1
  v/1 -> Product2/1
  Discrete-Time Integrator1/1 -> theta/1, sin(theta)/1, cos(theta)/1
  Product/1 -> Discrete-Time Integrator/1
  cos(theta)/1 -> Product/2
  Product2/1 -> Product/1, Product1/1
  sin(theta)/1 -> Product1/2
  Constant3/1 -> Discrete-Time Integrator/2
  Constant1/1 -> Discrete-Time Integrator1/2
  Constant2/1 -> Product2/2
  Discrete-Time Integrator/1 -> x/1
  Product1/1 -> Discrete-Time Integrator2/1
  Discrete-Time Integrator2/1 -> y/1
  Constant/1 -> Discrete-Time Integrator2/2

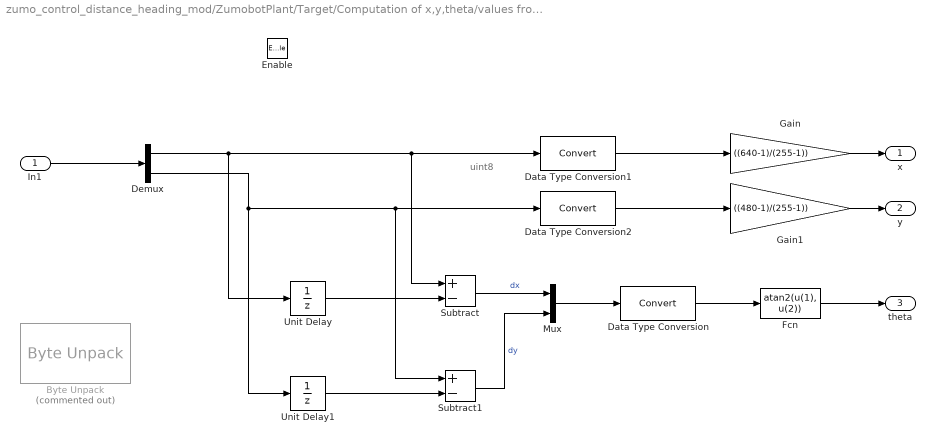
== system zumo_control_distance_heading_mod/ZumobotPlant/Target/Computation of x,y,theta/values from bluetooth /Subsystem ==
  note: uint8
  In1 : Inport
  Enable : EnablePort
  Byte Unpack : etargetslib/Byte Unpack  Commented=on  dimensions={1,1}  datatypes={'uint16', 'uint16'}  byteAlign=1
  Data Type Conversion : DataTypeConversion
  Data Type Conversion1 : DataTypeConversion
  Data Type Conversion2 : DataTypeConversion
  Demux : Demux  Outputs=2
  Fcn : Fcn  Expr=atan2(u(1), u(2))
  Gain : Gain  Gain=((640-1)/(255-1))
  Gain1 : Gain  Gain=((480-1)/(255-1))
  Mux : Mux  Inputs=2
  Subtract : Sum  Inputs=+-
  Subtract1 : Sum  Inputs=+-
  Unit Delay : UnitDelay  SampleTime=-1
  Unit Delay1 : UnitDelay  SampleTime=-1
  x : Outport  InitialOutput=150
  y : Outport  Port=2  InitialOutput=150
  theta : Outport  Port=3
  wires:
  Demux/1 -> Unit Delay/1, Data Type Conversion1/1, Subtract/1
  Demux/2 -> Unit Delay1/1, Data Type Conversion2/1, Subtract1/1
  Subtract1/1 -> Mux/2  "dy"
  Mux/1 -> Data Type Conversion/1
  Subtract/1 -> Mux/1  "dx"
  Fcn/1 -> theta/1
  Unit Delay/1 -> Subtract/2
  Unit Delay1/1 -> Subtract1/2
  In1/1 -> Demux/1
  Data Type Conversion/1 -> Fcn/1
  Data Type Conversion1/1 -> Gain/1
  Data Type Conversion2/1 -> Gain1/1
  Gain/1 -> x/1
  Gain1/1 -> y/1

== system zumo_control_distance_heading_mod/ZumobotPlant/Target/Computation of x,y,theta/values from bluetooth /Subsystem1 ==
  In1 : Inport
  Enable : EnablePort
  MATLAB Function : MATLAB Function  TreatAsAtomicUnit=on
  Out1 : Outport
  status : Outport  Port=2
  wires:
  In1/1 -> MATLAB Function/1(u)
  MATLAB Function/1(y) -> Out1/1
  MATLAB Function/2(trigger) -> status/1

== matlab function zumo_control_distance_heading_mod/ZumobotPlant/Target/Computation of x,y,theta/values from bluetooth /Subsystem1/MATLAB Function ==
  data: u input; y output; trigger output
function [y,trigger] = fcn(u)
%#codegen
persistent data count
if isempty(data)
    data = zeros(2,1,'uint8');
    count = 1;
end
trigger = 0;
data(count) = u;
count = count + 1;
if count > 2
    trigger = 1;
    count = 1;
end

y = data;

== matlab function zumo_control_distance_heading_mod/Controller/Subsystem/MATLAB Function ==
  data: previousReading input; deltaReading output; currentReading input; counter input
function deltaReading = handle360jump(previousReading, currentReading, counter)
%#codegen
deltaReading = 0;
if counter
    deltaReading = currentReading - previousReading;
    if abs(deltaReading) > 300
        if deltaReading > 0
            deltaReading = 360 - currentReading + previousReading;
        else
            deltaReading = 360 + deltaReading;
        end
    end
end
deltaReading = abs(deltaReading);

== matlab function zumo_control_distance_heading_mod/ZumobotPlant/Simulation/Computation of x,y,theta/values from bluetooth /Subsystem1/MATLAB Function ==
  data: u input; y output; trigger output
function [y,trigger] = fcn(u)
%#codegen
persistent data count
if isempty(data)
    data = zeros(4,1,'uint8');
    count = 1;
end
trigger = 0;
data(count) = u;
count = count + 1;
if count > 4
    trigger = 1;
    count = 1;
end

y = data;

== matlab function zumo_control_distance_heading_mod/Controller/Variant Subsystem/wmr ==
  data: X input; v output; Y input; DesiredX input; DesiredY input; DesiredHeading input; Heading input; omega output
function [v, omega] = wmr(X,Y,DesiredX,DesiredY,DesiredHeading, Heading)
%#codegen
% This function expects the dstates to be the difference of 
% dx = x_curr - x_dest; dy = y_curr - y_dest; dth = th_curr - th_dest;
persistent flag_initialize v_temp
if isempty(flag_initialize)
    flag_initialize = 1;
end
if isempty(v_temp)
    v_temp = 0;
end

dx = X - DesiredX;% cm
dy = Y - DesiredY;% cm
dth_degrees = Heading - DesiredHeading;% degrees (between 0 - 360)
dth = dth_degrees * pi/180; %in radians

dist_res = 1; %cm
heading_res = 5; %degrees
kp1 = 2;
kp2 = 12;
kd1 = 3;
kd2 = 7;
dt = 0.01;

if norm([dx dy]) < dist_res
    v = 0; %cm/s
    v_out = 0;
    if abs(dth_degrees) < heading_res
        omega = 0;%rad/s
    else
        omega = 360;%deg/s
    end
    %disp('Returning early.');
    return;
end
%% 
cth = cos(dth);
sth = sin(dth);

%% region division
region = 0; % initialize region
if dx >= 0 && dy >= 0     % add
    region = 1;
elseif dx < 0 && dy >= 0  % sugar
    region = 2;
elseif dx < 0 && dy < 0   % to
    region = 3;
elseif dx >= 0 && dy < 0  % coffee
    region = 4;
else
    error('Bad region: should not be here.');
end
%% region based inputs
if flag_initialize
    if region == 2 || region == 3
        v_temp = 32; %min threshold
    else % region = 1 || 4
        v_temp = -32; %min threshold
    end
    flag_initialize = 0;
end
% omega = 0;
%% computing v and omega 
v = v_temp;
v_out = v_temp;
xd = v*cth;
yd = v*sth;

u1 = -kp1*dx - kd1*xd;
u2 = -kp2*dy - kd2*yd;

v_temp = v_temp + (u1*cth + u2*sth) * dt; % cm/s
% v_prime = v_temp;
% saturate v_prime to a max of +255/-256 cm/s
% if v_prime > 255
%     v_prime = 255;
% elseif v_prime < -256
%     v_prime = -256;
% elseif v_prime < 32 && v_prime >= 0
%     v_prime = 32;
%     v_temp = v_prime;
% elseif v_prime > -32 && v_prime < 0
%     v_prime = -32;
%     v_temp = v_prime;
% end
v_tild = v_temp;
dvel = 5;
if abs(v_tild) < dvel
    v_tild = dvel;
%     v_temp = v_tild;
end

omega_rad_s = (u2*cth - u1*sth)/(v_tild); %rad/s

% convert rad/s into deg/s (as the plant model accepts that)
omega = omega_rad_s * (180/pi);

% % maximum omega(rad/s) allowed = ~2*pi/sec
% if omega > 360
%     omega= 360;
% elseif omega < -360
%     omega = -360;
% end

== matlab function zumo_control_distance_heading_mod/Controller/Variant Subsystem/controllyap ==
  data: X input; v output; Y input; DesiredX input; DesiredY input; DesiredHeading input; Heading input; omega output
function [v, omega] = controllyap(X,Y,DesiredX,DesiredY,DesiredHeading,Heading)

persistent th_mag_north R_mc
heading = Heading*pi/180;
if isempty(th_mag_north)
    th_mag_north = heading;
    % magnetic north wrt to camera frame: we have to align the robot to the
    % camera frame at the start
    R_mc = [cos(-heading),-sin(-heading);sin(-heading),cos(-heading)] * [1 0;0 -1];
end
% current robot frame wrt magnetic frame
R_rm = [cos(heading),-sin(heading);sin(heading),cos(heading)]; 
% destination frame wrt magnetic frame
d_heading = DesiredHeading*pi/180;
R_dm = [cos(d_heading),-sin(d_heading);sin(d_heading),cos(d_heading)];
% observations : 
% 1. if the error is ~130 in both x,y, direction the controller
% is working fine

% in camera frame
dx_c =-(X - DesiredX);% cm
dy_c = -(Y - DesiredY);% cm

% % % in current robot frame
% % d_r = R_rm*R_mc*[dx;dy];
% % dx_r = d_r(1);
% % dy_r = d_r(2);

% in destination robot frame
d_d = R_dm*R_mc*[dx_c;dy_c];
dx_d = d_d(1);
dy_d = d_d(2);

phi_des = DesiredHeading*pi/180;

%% computing phi
phi_deg = (Heading - th_mag_north*180/pi);
if 180<phi_deg
    phi_deg = -phi_deg+360;
elseif phi_deg<-180
    phi_deg = phi_deg+360;
end
phi = phi_deg*pi/180;
%phi = Heading;
%% error computation in desired frame
e = sqrt(dx_d^2+dy_d^2);

% if e < 4
%     v = 0;
%     omega = 0;
%     return;
% end
% dir = [cos(phi_des),sin(phi_des)];
% ang = atan2(sin(phi_des),cos(phi_des));
ang = (phi_des -  th_mag_north); % radians
temp = atan2(dy_d,dx_d);
if temp <-pi
   temp = temp+2*pi; 
end;

theta = temp-ang;
alpha = temp-phi;

%if pi<alpha
%    alpha = alpha-2*pi;
%elseif alpha<-pi%    
%    alpha =alpha+2*pi;
%end

gamma = 1;
k = 2;
h = 2;
% dist_res = .01; %cm
% heading_res = 1; %degrees

%% compute the controller v and omega
omega = k*alpha+gamma*((cos(alpha)*sin(alpha))/alpha)*(alpha+h*theta);
if isnan(omega)
    omega = pi;
end
v =  cos(alpha)*e*gamma;

%% convert omega (deg/s -> rad/s)
omega = omega * (180/pi);

%% throttling the velocity so that zumo moves slowly.
v_threshold = 15;

if abs(v) > v_threshold
    v = sign(v)*v_threshold;
end

% omega_threshold = 90;
% 
% if abs(omega) > omega_threshold
%     omega = sign(omega)*omega_threshold;
%     
% end

%% hitting convergence
if e < 20
        v = 0;
        omega = 0;
end 
% if abs(phi-phi_des)<5*pi/180 || v == 0      
%     omega = 0;
% end

== matlab function zumo_control_distance_heading_mod/Controller/Variant Subsystem/PrimitiveControl/TurnTowardsDestination/Compute ==
  data: X input; destinationDirection output; Y input; DesiredX input; DesiredY input; Heading input
function destinationDirection = computeFirstHeadingChange(X,Y,DesiredX,DesiredY,Heading)
%#codegen
persistent th_mag_north R_mc

heading = Heading*pi/180;
if isempty(th_mag_north)
    % as we allign robot's x (forward) towards camera's x direction
    % hence the initial heading is : where the robot frame is wrt magentic
    % north
    % Now, as we oriented robot with camera frame, it is also the camera
    % frame wrt magentic north (at that heading angle)
    th_mag_north = heading;
    R_mc = RotZ(-th_mag_north)*[1 0;0 -1]; %R_magneticNorth_wrt_CameraFrame
end

% in camera frame
dx_c = DesiredX - X;
dy_c = DesiredY - Y;

%in magnetic north frame
d_m = R_mc * [dx_c;dy_c];
dx_m = d_m(1);
dy_m = d_m(2);

% if dx_m == 0 && dy_m ==0
%     % if at th start it is at the destination, then dont move
%     destinationDirection = heading;
% else
    destinationDirection = atan2(dy_m, dx_m); %in magnetic north frame

    % atan2 gives output in (-pi, pi)
    if destinationDirection < 0
        destinationDirection = destinationDirection + 2*pi;
    end
    % now destinationDirection is in (0,2pi)
% end

destinationDirection = destinationDirection*180/pi; %in degrees
end

function rotationMatrix = RotZ(th)
    sth = sin(th);
    cth = cos(th);
    rotationMatrix = [cth -sth; sth cth];
end
